simulink model "comparing_controllers"  (R2020a)
settings: Solver=VariableStepAuto  StartTime=0.0  StopTime=50  RelTol=1e-3
libraries: aerolibutil x20, sharedutil x10, slctrlblks x6
(part 2 of 3)

== system comparing_controllers/PD Gravity Compensated Controller/6 DOF PD Gravity Comp Controller/Subsystem3/Subsystem1 ==
  NED : Inport
  Demux : Demux  Outputs=2
  Demux1 : Demux  Outputs=3
  Derivative : Derivative  Commented=on
  Invert 3x3 Matrix : aerolibutil/Invert  3x3 Matrix
  Invert 3x3 Matrix1 : aerolibutil/Invert  3x3 Matrix  Commented=on
  MatrixMultiply : Product  Commented=on  Multiplication=Matrix(*)
  MatrixMultiply1 : Product  Multiplication=Matrix(*)
  Mux1 : Mux  Inputs=3
  Rzxy : Subsystem
  T : Subsystem  Commented=on
  Terminator : Terminator  Commented=on
  pos_body : Outport
  wires:
  Demux1/2 -> Mux1/2, T/2(In2)  "theta"
  Demux1/1 -> Mux1/1, T/1(In1)  "phi"
  Rzxy/1(J) -> Invert 3x3 Matrix/1
  Mux1/1 -> Derivative/1, Rzxy/1(angles)
  Derivative/1 -> MatrixMultiply/2  "euler_dot"
  Invert 3x3 Matrix1/1 -> MatrixMultiply/1  "T'"
  Demux1/3 -> Mux1/3  "psi"
  MatrixMultiply/1 -> Terminator/1  "ang_vel_body"
  T/1(T) -> Invert 3x3 Matrix1/1
  Invert 3x3 Matrix/1 -> MatrixMultiply1/1  "R'"
  MatrixMultiply1/1 -> pos_body/1
  NED/1 -> Demux/1
  Demux/2 -> Demux1/1
  Demux/1 -> MatrixMultiply1/2

== system comparing_controllers/PD Gravity Compensated Controller/6 DOF PD Gravity Comp Controller/Subsystem3/Subsystem2 ==
  NED : Inport
  Demux : Demux  Outputs=2
  Demux1 : Demux  Outputs=3
  Derivative : Derivative  Commented=on
  Invert 3x3 Matrix : aerolibutil/Invert  3x3 Matrix
  Invert 3x3 Matrix1 : aerolibutil/Invert  3x3 Matrix  Commented=on
  MatrixMultiply : Product  Commented=on  Multiplication=Matrix(*)
  MatrixMultiply1 : Product  Multiplication=Matrix(*)
  Mux1 : Mux  Inputs=3
  Rzxy : Subsystem
  T : Subsystem  Commented=on
  Terminator : Terminator  Commented=on
  pos_body : Outport
  wires:
  Demux1/2 -> Mux1/2, T/2(In2)  "theta"
  Demux1/1 -> Mux1/1, T/1(In1)  "phi"
  Rzxy/1(J) -> Invert 3x3 Matrix/1
  Mux1/1 -> Derivative/1, Rzxy/1(angles)
  Derivative/1 -> MatrixMultiply/2  "euler_dot"
  Invert 3x3 Matrix1/1 -> MatrixMultiply/1  "T'"
  Demux1/3 -> Mux1/3  "psi"
  MatrixMultiply/1 -> Terminator/1  "ang_vel_body"
  T/1(T) -> Invert 3x3 Matrix1/1
  Invert 3x3 Matrix/1 -> MatrixMultiply1/1  "R'"
  MatrixMultiply1/1 -> pos_body/1
  NED/1 -> Demux/1
  Demux/2 -> Demux1/1
  Demux/1 -> MatrixMultiply1/2

== system comparing_controllers/PD Gravity Compensated Controller/6 DOF PD Gravity Comp Controller/Transform/Subsystem1 ==
  NED : Inport
  Demux : Demux  Outputs=2
  Demux1 : Demux  Outputs=3
  Derivative : Derivative  Commented=on
  Invert 3x3 Matrix : aerolibutil/Invert  3x3 Matrix
  Invert 3x3 Matrix1 : aerolibutil/Invert  3x3 Matrix  Commented=on
  MatrixMultiply : Product  Commented=on  Multiplication=Matrix(*)
  MatrixMultiply1 : Product  Multiplication=Matrix(*)
  Mux1 : Mux  Inputs=3
  Rzxy : Subsystem
  T : Subsystem  Commented=on
  Terminator : Terminator  Commented=on
  pos_body : Outport
  wires:
  Demux1/2 -> Mux1/2, T/2(In2)  "theta"
  Demux1/1 -> Mux1/1, T/1(In1)  "phi"
  Rzxy/1(J) -> Invert 3x3 Matrix/1
  Mux1/1 -> Derivative/1, Rzxy/1(angles)
  Derivative/1 -> MatrixMultiply/2  "euler_dot"
  Invert 3x3 Matrix1/1 -> MatrixMultiply/1  "T'"
  Demux1/3 -> Mux1/3  "psi"
  MatrixMultiply/1 -> Terminator/1  "ang_vel_body"
  T/1(T) -> Invert 3x3 Matrix1/1
  Invert 3x3 Matrix/1 -> MatrixMultiply1/1  "R'"
  MatrixMultiply1/1 -> pos_body/1
  NED/1 -> Demux/1
  Demux/2 -> Demux1/1
  Demux/1 -> MatrixMultiply1/2

== system comparing_controllers/PD Gravity Compensated Controller/6 DOF PD Gravity Comp Controller/Transform/Subsystem2 ==
  NED : Inport
  Demux : Demux  Outputs=2
  Demux1 : Demux  Outputs=3
  Derivative : Derivative  Commented=on
  Invert 3x3 Matrix : aerolibutil/Invert  3x3 Matrix
  Invert 3x3 Matrix1 : aerolibutil/Invert  3x3 Matrix  Commented=on
  MatrixMultiply : Product  Commented=on  Multiplication=Matrix(*)
  MatrixMultiply1 : Product  Multiplication=Matrix(*)
  Mux1 : Mux  Inputs=3
  Rzxy : Subsystem
  T : Subsystem  Commented=on
  Terminator : Terminator  Commented=on
  pos_body : Outport
  wires:
  Demux1/2 -> Mux1/2, T/2(In2)  "theta"
  Demux1/1 -> Mux1/1, T/1(In1)  "phi"
  Rzxy/1(J) -> Invert 3x3 Matrix/1
  Mux1/1 -> Derivative/1, Rzxy/1(angles)
  Derivative/1 -> MatrixMultiply/2  "euler_dot"
  Invert 3x3 Matrix1/1 -> MatrixMultiply/1  "T'"
  Demux1/3 -> Mux1/3  "psi"
  MatrixMultiply/1 -> Terminator/1  "ang_vel_body"
  T/1(T) -> Invert 3x3 Matrix1/1
  Invert 3x3 Matrix/1 -> MatrixMultiply1/1  "R'"
  MatrixMultiply1/1 -> pos_body/1
  NED/1 -> Demux/1
  Demux/2 -> Demux1/1
  Demux/1 -> MatrixMultiply1/2

== system comparing_controllers/PID Controller/6 DOF PID Controller/Transform/Subsystem1 ==
  NED : Inport
  Demux : Demux  Outputs=2
  Demux1 : Demux  Outputs=3
  Derivative : Derivative  Commented=on
  Invert 3x3 Matrix : aerolibutil/Invert  3x3 Matrix
  Invert 3x3 Matrix1 : aerolibutil/Invert  3x3 Matrix  Commented=on
  MatrixMultiply : Product  Commented=on  Multiplication=Matrix(*)
  MatrixMultiply1 : Product  Multiplication=Matrix(*)
  Mux1 : Mux  Inputs=3
  Rzxy : Subsystem
  T : Subsystem  Commented=on
  Terminator : Terminator  Commented=on
  pos_body : Outport
  wires:
  Demux1/2 -> Mux1/2, T/2(In2)  "theta"
  Demux1/1 -> Mux1/1, T/1(In1)  "phi"
  Rzxy/1(J) -> Invert 3x3 Matrix/1
  Mux1/1 -> Derivative/1, Rzxy/1(angles)
  Derivative/1 -> MatrixMultiply/2  "euler_dot"
  Invert 3x3 Matrix1/1 -> MatrixMultiply/1  "T'"
  Demux1/3 -> Mux1/3  "psi"
  MatrixMultiply/1 -> Terminator/1  "ang_vel_body"
  T/1(T) -> Invert 3x3 Matrix1/1
  Invert 3x3 Matrix/1 -> MatrixMultiply1/1  "R'"
  MatrixMultiply1/1 -> pos_body/1
  NED/1 -> Demux/1
  Demux/2 -> Demux1/1
  Demux/1 -> MatrixMultiply1/2

== system comparing_controllers/PID Controller/6 DOF PID Controller/Transform/Subsystem2 ==
  NED : Inport
  Demux : Demux  Outputs=2
  Demux1 : Demux  Outputs=3
  Derivative : Derivative  Commented=on
  Invert 3x3 Matrix : aerolibutil/Invert  3x3 Matrix
  Invert 3x3 Matrix1 : aerolibutil/Invert  3x3 Matrix  Commented=on
  MatrixMultiply : Product  Commented=on  Multiplication=Matrix(*)
  MatrixMultiply1 : Product  Multiplication=Matrix(*)
  Mux1 : Mux  Inputs=3
  Rzxy : Subsystem
  T : Subsystem  Commented=on
  Terminator : Terminator  Commented=on
  pos_body : Outport
  wires:
  Demux1/2 -> Mux1/2, T/2(In2)  "theta"
  Demux1/1 -> Mux1/1, T/1(In1)  "phi"
  Rzxy/1(J) -> Invert 3x3 Matrix/1
  Mux1/1 -> Derivative/1, Rzxy/1(angles)
  Derivative/1 -> MatrixMultiply/2  "euler_dot"
  Invert 3x3 Matrix1/1 -> MatrixMultiply/1  "T'"
  Demux1/3 -> Mux1/3  "psi"
  MatrixMultiply/1 -> Terminator/1  "ang_vel_body"
  T/1(T) -> Invert 3x3 Matrix1/1
  Invert 3x3 Matrix/1 -> MatrixMultiply1/1  "R'"
  MatrixMultiply1/1 -> pos_body/1
  NED/1 -> Demux/1
  Demux/2 -> Demux1/1
  Demux/1 -> MatrixMultiply1/2

== system comparing_controllers/Computed Torque/Computed Torque Controller/Transform/Subsystem1/Rzxy ==
  angles : Inport
  3-2-1 convention : Product  Inputs=3  Multiplication=Matrix(*)
  Demux : Demux  Outputs=3
  MATLAB Function1 : MATLAB Function  TreatAsAtomicUnit=on
  MATLAB Function2 : MATLAB Function  TreatAsAtomicUnit=on
  MATLAB Function3 : MATLAB Function  TreatAsAtomicUnit=on
  J : Outport
  wires:
  Demux/1 -> MATLAB Function1/1(phi)
  MATLAB Function3/1(Rz) -> 3-2-1 convention/1
  MATLAB Function2/1(Ry) -> 3-2-1 convention/2
  Demux/3 -> MATLAB Function3/1(psi)
  MATLAB Function1/1(Rx) -> 3-2-1 convention/3
  3-2-1 convention/1 -> J/1
  angles/1 -> Demux/1
  Demux/2 -> MATLAB Function2/1(theta)

== system comparing_controllers/Computed Torque/Computed Torque Controller/Transform/Subsystem1/T ==
  In1 : Inport
  In2 : Inport  Port=2
  Constant1 : Constant
  Constant2 : Constant  Value=0
  Create 3x3 Matrix : sharedutil/Create 3x3 Matrix  aMode=aMode
      settings: SourceProductBaseCode=AE,PW,MT,VE,VP
  Divide : Product  Inputs=*/
  Divide1 : Product  Inputs=*/
  Gain : Gain  Gain=-1
  Product : Product
  Product1 : Product
  Sin : Trigonometry
  Sin1 : Trigonometry  Operator=cos
  Sin2 : Trigonometry  Operator=tan
  Sin3 : Trigonometry  Operator=cos
  T : Outport
  wires:
  Constant2/1 -> Create 3x3 Matrix/7, Create 3x3 Matrix/4
  Create 3x3 Matrix/1 -> T/1
  Gain/1 -> Create 3x3 Matrix/6
  Divide1/1 -> Create 3x3 Matrix/9
  Product/1 -> Create 3x3 Matrix/2
  Sin1/1 -> Divide1/1, Create 3x3 Matrix/5, Product1/1
  In1/1 -> Sin1/1, Sin/1  "phi"
  Sin2/1 -> Product/2, Product1/2
  Divide/1 -> Create 3x3 Matrix/8
  Product1/1 -> Create 3x3 Matrix/3
  Sin3/1 -> Divide1/2, Divide/2
  In2/1 -> Sin2/1, Sin3/1  "theta"
  Sin/1 -> Gain/1, Divide/1, Product/1
  Constant1/1 -> Create 3x3 Matrix/1

== system comparing_controllers/Computed Torque/Computed Torque Controller/Transform/Subsystem2/Rzxy ==
  angles : Inport
  3-2-1 convention : Product  Inputs=3  Multiplication=Matrix(*)
  Demux : Demux  Outputs=3
  MATLAB Function1 : MATLAB Function  TreatAsAtomicUnit=on
  MATLAB Function2 : MATLAB Function  TreatAsAtomicUnit=on
  MATLAB Function3 : MATLAB Function  TreatAsAtomicUnit=on
  J : Outport
  wires:
  Demux/1 -> MATLAB Function1/1(phi)
  MATLAB Function3/1(Rz) -> 3-2-1 convention/1
  MATLAB Function2/1(Ry) -> 3-2-1 convention/2
  Demux/3 -> MATLAB Function3/1(psi)
  MATLAB Function1/1(Rx) -> 3-2-1 convention/3
  3-2-1 convention/1 -> J/1
  angles/1 -> Demux/1
  Demux/2 -> MATLAB Function2/1(theta)

== system comparing_controllers/Computed Torque/Computed Torque Controller/Transform/Subsystem2/T ==
  In1 : Inport
  In2 : Inport  Port=2
  Constant1 : Constant
  Constant2 : Constant  Value=0
  Create 3x3 Matrix : sharedutil/Create 3x3 Matrix  aMode=aMode
      settings: SourceProductBaseCode=AE,PW,MT,VE,VP
  Divide : Product  Inputs=*/
  Divide1 : Product  Inputs=*/
  Gain : Gain  Gain=-1
  Product : Product
  Product1 : Product
  Sin : Trigonometry
  Sin1 : Trigonometry  Operator=cos
  Sin2 : Trigonometry  Operator=tan
  Sin3 : Trigonometry  Operator=cos
  T : Outport
  wires:
  Constant2/1 -> Create 3x3 Matrix/7, Create 3x3 Matrix/4
  Create 3x3 Matrix/1 -> T/1
  Gain/1 -> Create 3x3 Matrix/6
  Divide1/1 -> Create 3x3 Matrix/9
  Product/1 -> Create 3x3 Matrix/2
  Sin1/1 -> Divide1/1, Create 3x3 Matrix/5, Product1/1
  In1/1 -> Sin1/1, Sin/1  "phi"
  Sin2/1 -> Product/2, Product1/2
  Divide/1 -> Create 3x3 Matrix/8
  Product1/1 -> Create 3x3 Matrix/3
  Sin3/1 -> Divide1/2, Divide/2
  In2/1 -> Sin2/1, Sin3/1  "theta"
  Sin/1 -> Gain/1, Divide/1, Product/1
  Constant1/1 -> Create 3x3 Matrix/1

== system comparing_controllers/PD Controller/6 DOF PD Controller/Transform/Subsystem1/Rzxy ==
  angles : Inport
  3-2-1 convention : Product  Inputs=3  Multiplication=Matrix(*)
  Demux : Demux  Outputs=3
  MATLAB Function1 : MATLAB Function  TreatAsAtomicUnit=on
  MATLAB Function2 : MATLAB Function  TreatAsAtomicUnit=on
  MATLAB Function3 : MATLAB Function  TreatAsAtomicUnit=on
  J : Outport
  wires:
  Demux/1 -> MATLAB Function1/1(phi)
  MATLAB Function3/1(Rz) -> 3-2-1 convention/1
  MATLAB Function2/1(Ry) -> 3-2-1 convention/2
  Demux/3 -> MATLAB Function3/1(psi)
  MATLAB Function1/1(Rx) -> 3-2-1 convention/3
  3-2-1 convention/1 -> J/1
  angles/1 -> Demux/1
  Demux/2 -> MATLAB Function2/1(theta)

== system comparing_controllers/PD Controller/6 DOF PD Controller/Transform/Subsystem1/T ==
  In1 : Inport
  In2 : Inport  Port=2
  Constant1 : Constant
  Constant2 : Constant  Value=0
  Create 3x3 Matrix : sharedutil/Create 3x3 Matrix  aMode=aMode
      settings: SourceProductBaseCode=AE,PW,MT,VE,VP
  Divide : Product  Inputs=*/
  Divide1 : Product  Inputs=*/
  Gain : Gain  Gain=-1
  Product : Product
  Product1 : Product
  Sin : Trigonometry
  Sin1 : Trigonometry  Operator=cos
  Sin2 : Trigonometry  Operator=tan
  Sin3 : Trigonometry  Operator=cos
  T : Outport
  wires:
  Constant2/1 -> Create 3x3 Matrix/7, Create 3x3 Matrix/4
  Create 3x3 Matrix/1 -> T/1
  Gain/1 -> Create 3x3 Matrix/6
  Divide1/1 -> Create 3x3 Matrix/9
  Product/1 -> Create 3x3 Matrix/2
  Sin1/1 -> Divide1/1, Create 3x3 Matrix/5, Product1/1
  In1/1 -> Sin1/1, Sin/1  "phi"
  Sin2/1 -> Product/2, Product1/2
  Divide/1 -> Create 3x3 Matrix/8
  Product1/1 -> Create 3x3 Matrix/3
  Sin3/1 -> Divide1/2, Divide/2
  In2/1 -> Sin2/1, Sin3/1  "theta"
  Sin/1 -> Gain/1, Divide/1, Product/1
  Constant1/1 -> Create 3x3 Matrix/1

== system comparing_controllers/PD Controller/6 DOF PD Controller/Transform/Subsystem2/Rzxy ==
  angles : Inport
  3-2-1 convention : Product  Inputs=3  Multiplication=Matrix(*)
  Demux : Demux  Outputs=3
  MATLAB Function1 : MATLAB Function  TreatAsAtomicUnit=on
  MATLAB Function2 : MATLAB Function  TreatAsAtomicUnit=on
  MATLAB Function3 : MATLAB Function  TreatAsAtomicUnit=on
  J : Outport
  wires:
  Demux/1 -> MATLAB Function1/1(phi)
  MATLAB Function3/1(Rz) -> 3-2-1 convention/1
  MATLAB Function2/1(Ry) -> 3-2-1 convention/2
  Demux/3 -> MATLAB Function3/1(psi)
  MATLAB Function1/1(Rx) -> 3-2-1 convention/3
  3-2-1 convention/1 -> J/1
  angles/1 -> Demux/1
  Demux/2 -> MATLAB Function2/1(theta)

== system comparing_controllers/PD Controller/6 DOF PD Controller/Transform/Subsystem2/T ==
  In1 : Inport
  In2 : Inport  Port=2
  Constant1 : Constant
  Constant2 : Constant  Value=0
  Create 3x3 Matrix : sharedutil/Create 3x3 Matrix  aMode=aMode
      settings: SourceProductBaseCode=AE,PW,MT,VE,VP
  Divide : Product  Inputs=*/
  Divide1 : Product  Inputs=*/
  Gain : Gain  Gain=-1
  Product : Product
  Product1 : Product
  Sin : Trigonometry
  Sin1 : Trigonometry  Operator=cos
  Sin2 : Trigonometry  Operator=tan
  Sin3 : Trigonometry  Operator=cos
  T : Outport
  wires:
  Constant2/1 -> Create 3x3 Matrix/7, Create 3x3 Matrix/4
  Create 3x3 Matrix/1 -> T/1
  Gain/1 -> Create 3x3 Matrix/6
  Divide1/1 -> Create 3x3 Matrix/9
  Product/1 -> Create 3x3 Matrix/2
  Sin1/1 -> Divide1/1, Create 3x3 Matrix/5, Product1/1
  In1/1 -> Sin1/1, Sin/1  "phi"
  Sin2/1 -> Product/2, Product1/2
  Divide/1 -> Create 3x3 Matrix/8
  Product1/1 -> Create 3x3 Matrix/3
  Sin3/1 -> Divide1/2, Divide/2
  In2/1 -> Sin2/1, Sin3/1  "theta"
  Sin/1 -> Gain/1, Divide/1, Product/1
  Constant1/1 -> Create 3x3 Matrix/1

== system comparing_controllers/PD Gravity Compensated Controller/6 DOF PD Gravity Comp Controller/Subsystem3/Subsystem1/Rzxy ==
  angles : Inport
  3-2-1 convention : Product  Inputs=3  Multiplication=Matrix(*)
  Demux : Demux  Outputs=3
  MATLAB Function1 : MATLAB Function  TreatAsAtomicUnit=on
  MATLAB Function2 : MATLAB Function  TreatAsAtomicUnit=on
  MATLAB Function3 : MATLAB Function  TreatAsAtomicUnit=on
  J : Outport
  wires:
  Demux/1 -> MATLAB Function1/1(phi)
  MATLAB Function3/1(Rz) -> 3-2-1 convention/1
  MATLAB Function2/1(Ry) -> 3-2-1 convention/2
  Demux/3 -> MATLAB Function3/1(psi)
  MATLAB Function1/1(Rx) -> 3-2-1 convention/3
  3-2-1 convention/1 -> J/1
  angles/1 -> Demux/1
  Demux/2 -> MATLAB Function2/1(theta)

== system comparing_controllers/PD Gravity Compensated Controller/6 DOF PD Gravity Comp Controller/Subsystem3/Subsystem1/T ==
  In1 : Inport
  In2 : Inport  Port=2
  Constant1 : Constant
  Constant2 : Constant  Value=0
  Create 3x3 Matrix : sharedutil/Create 3x3 Matrix  aMode=aMode
      settings: SourceProductBaseCode=AE,PW,MT,VE,VP
  Divide : Product  Inputs=*/
  Divide1 : Product  Inputs=*/
  Gain : Gain  Gain=-1
  Product : Product
  Product1 : Product
  Sin : Trigonometry
  Sin1 : Trigonometry  Operator=cos
  Sin2 : Trigonometry  Operator=tan
  Sin3 : Trigonometry  Operator=cos
  T : Outport
  wires:
  Constant2/1 -> Create 3x3 Matrix/7, Create 3x3 Matrix/4
  Create 3x3 Matrix/1 -> T/1
  Gain/1 -> Create 3x3 Matrix/6
  Divide1/1 -> Create 3x3 Matrix/9
  Product/1 -> Create 3x3 Matrix/2
  Sin1/1 -> Divide1/1, Create 3x3 Matrix/5, Product1/1
  In1/1 -> Sin1/1, Sin/1  "phi"
  Sin2/1 -> Product/2, Product1/2
  Divide/1 -> Create 3x3 Matrix/8
  Product1/1 -> Create 3x3 Matrix/3
  Sin3/1 -> Divide1/2, Divide/2
  In2/1 -> Sin2/1, Sin3/1  "theta"
  Sin/1 -> Gain/1, Divide/1, Product/1
  Constant1/1 -> Create 3x3 Matrix/1

== system comparing_controllers/PD Gravity Compensated Controller/6 DOF PD Gravity Comp Controller/Subsystem3/Subsystem2/Rzxy ==
  angles : Inport
  3-2-1 convention : Product  Inputs=3  Multiplication=Matrix(*)
  Demux : Demux  Outputs=3
  MATLAB Function1 : MATLAB Function  TreatAsAtomicUnit=on
  MATLAB Function2 : MATLAB Function  TreatAsAtomicUnit=on
  MATLAB Function3 : MATLAB Function  TreatAsAtomicUnit=on
  J : Outport
  wires:
  Demux/1 -> MATLAB Function1/1(phi)
  MATLAB Function3/1(Rz) -> 3-2-1 convention/1
  MATLAB Function2/1(Ry) -> 3-2-1 convention/2
  Demux/3 -> MATLAB Function3/1(psi)
  MATLAB Function1/1(Rx) -> 3-2-1 convention/3
  3-2-1 convention/1 -> J/1
  angles/1 -> Demux/1
  Demux/2 -> MATLAB Function2/1(theta)

== system comparing_controllers/PD Gravity Compensated Controller/6 DOF PD Gravity Comp Controller/Subsystem3/Subsystem2/T ==
  In1 : Inport
  In2 : Inport  Port=2
  Constant1 : Constant
  Constant2 : Constant  Value=0
  Create 3x3 Matrix : sharedutil/Create 3x3 Matrix  aMode=aMode
      settings: SourceProductBaseCode=AE,PW,MT,VE,VP
  Divide : Product  Inputs=*/
  Divide1 : Product  Inputs=*/
  Gain : Gain  Gain=-1
  Product : Product
  Product1 : Product
  Sin : Trigonometry
  Sin1 : Trigonometry  Operator=cos
  Sin2 : Trigonometry  Operator=tan
  Sin3 : Trigonometry  Operator=cos
  T : Outport
  wires:
  Constant2/1 -> Create 3x3 Matrix/7, Create 3x3 Matrix/4
  Create 3x3 Matrix/1 -> T/1
  Gain/1 -> Create 3x3 Matrix/6
  Divide1/1 -> Create 3x3 Matrix/9
  Product/1 -> Create 3x3 Matrix/2
  Sin1/1 -> Divide1/1, Create 3x3 Matrix/5, Product1/1
  In1/1 -> Sin1/1, Sin/1  "phi"
  Sin2/1 -> Product/2, Product1/2
  Divide/1 -> Create 3x3 Matrix/8
  Product1/1 -> Create 3x3 Matrix/3
  Sin3/1 -> Divide1/2, Divide/2
  In2/1 -> Sin2/1, Sin3/1  "theta"
  Sin/1 -> Gain/1, Divide/1, Product/1
  Constant1/1 -> Create 3x3 Matrix/1

== system comparing_controllers/PD Gravity Compensated Controller/6 DOF PD Gravity Comp Controller/Transform/Subsystem1/Rzxy ==
  angles : Inport
  3-2-1 convention : Product  Inputs=3  Multiplication=Matrix(*)
  Demux : Demux  Outputs=3
  MATLAB Function1 : MATLAB Function  TreatAsAtomicUnit=on
  MATLAB Function2 : MATLAB Function  TreatAsAtomicUnit=on
  MATLAB Function3 : MATLAB Function  TreatAsAtomicUnit=on
  J : Outport
  wires:
  Demux/1 -> MATLAB Function1/1(phi)
  MATLAB Function3/1(Rz) -> 3-2-1 convention/1
  MATLAB Function2/1(Ry) -> 3-2-1 convention/2
  Demux/3 -> MATLAB Function3/1(psi)
  MATLAB Function1/1(Rx) -> 3-2-1 convention/3
  3-2-1 convention/1 -> J/1
  angles/1 -> Demux/1
  Demux/2 -> MATLAB Function2/1(theta)

== system comparing_controllers/PD Gravity Compensated Controller/6 DOF PD Gravity Comp Controller/Transform/Subsystem1/T ==
  In1 : Inport
  In2 : Inport  Port=2
  Constant1 : Constant
  Constant2 : Constant  Value=0
  Create 3x3 Matrix : sharedutil/Create 3x3 Matrix  aMode=aMode
      settings: SourceProductBaseCode=AE,PW,MT,VE,VP
  Divide : Product  Inputs=*/
  Divide1 : Product  Inputs=*/
  Gain : Gain  Gain=-1
  Product : Product
  Product1 : Product
  Sin : Trigonometry
  Sin1 : Trigonometry  Operator=cos
  Sin2 : Trigonometry  Operator=tan
  Sin3 : Trigonometry  Operator=cos
  T : Outport
  wires:
  Constant2/1 -> Create 3x3 Matrix/7, Create 3x3 Matrix/4
  Create 3x3 Matrix/1 -> T/1
  Gain/1 -> Create 3x3 Matrix/6
  Divide1/1 -> Create 3x3 Matrix/9
  Product/1 -> Create 3x3 Matrix/2
  Sin1/1 -> Divide1/1, Create 3x3 Matrix/5, Product1/1
  In1/1 -> Sin1/1, Sin/1  "phi"
  Sin2/1 -> Product/2, Product1/2
  Divide/1 -> Create 3x3 Matrix/8
  Product1/1 -> Create 3x3 Matrix/3
  Sin3/1 -> Divide1/2, Divide/2
  In2/1 -> Sin2/1, Sin3/1  "theta"
  Sin/1 -> Gain/1, Divide/1, Product/1
  Constant1/1 -> Create 3x3 Matrix/1

== system comparing_controllers/PD Gravity Compensated Controller/6 DOF PD Gravity Comp Controller/Transform/Subsystem2/Rzxy ==
  angles : Inport
  3-2-1 convention : Product  Inputs=3  Multiplication=Matrix(*)
  Demux : Demux  Outputs=3
  MATLAB Function1 : MATLAB Function  TreatAsAtomicUnit=on
  MATLAB Function2 : MATLAB Function  TreatAsAtomicUnit=on
  MATLAB Function3 : MATLAB Function  TreatAsAtomicUnit=on
  J : Outport
  wires:
  Demux/1 -> MATLAB Function1/1(phi)
  MATLAB Function3/1(Rz) -> 3-2-1 convention/1
  MATLAB Function2/1(Ry) -> 3-2-1 convention/2
  Demux/3 -> MATLAB Function3/1(psi)
  MATLAB Function1/1(Rx) -> 3-2-1 convention/3
  3-2-1 convention/1 -> J/1
  angles/1 -> Demux/1
  Demux/2 -> MATLAB Function2/1(theta)

== system comparing_controllers/PD Gravity Compensated Controller/6 DOF PD Gravity Comp Controller/Transform/Subsystem2/T ==
  In1 : Inport
  In2 : Inport  Port=2
  Constant1 : Constant
  Constant2 : Constant  Value=0
  Create 3x3 Matrix : sharedutil/Create 3x3 Matrix  aMode=aMode
      settings: SourceProductBaseCode=AE,PW,MT,VE,VP
  Divide : Product  Inputs=*/
  Divide1 : Product  Inputs=*/
  Gain : Gain  Gain=-1
  Product : Product
  Product1 : Product
  Sin : Trigonometry
  Sin1 : Trigonometry  Operator=cos
  Sin2 : Trigonometry  Operator=tan
  Sin3 : Trigonometry  Operator=cos
  T : Outport
  wires:
  Constant2/1 -> Create 3x3 Matrix/7, Create 3x3 Matrix/4
  Create 3x3 Matrix/1 -> T/1
  Gain/1 -> Create 3x3 Matrix/6
  Divide1/1 -> Create 3x3 Matrix/9
  Product/1 -> Create 3x3 Matrix/2
  Sin1/1 -> Divide1/1, Create 3x3 Matrix/5, Product1/1
  In1/1 -> Sin1/1, Sin/1  "phi"
  Sin2/1 -> Product/2, Product1/2
  Divide/1 -> Create 3x3 Matrix/8
  Product1/1 -> Create 3x3 Matrix/3
  Sin3/1 -> Divide1/2, Divide/2
  In2/1 -> Sin2/1, Sin3/1  "theta"
  Sin/1 -> Gain/1, Divide/1, Product/1
  Constant1/1 -> Create 3x3 Matrix/1

== system comparing_controllers/PID Controller/6 DOF PID Controller/Transform/Subsystem1/Rzxy ==
  angles : Inport
  3-2-1 convention : Product  Inputs=3  Multiplication=Matrix(*)
  Demux : Demux  Outputs=3
  MATLAB Function1 : MATLAB Function  TreatAsAtomicUnit=on
  MATLAB Function2 : MATLAB Function  TreatAsAtomicUnit=on
  MATLAB Function3 : MATLAB Function  TreatAsAtomicUnit=on
  J : Outport
  wires:
  Demux/1 -> MATLAB Function1/1(phi)
  MATLAB Function3/1(Rz) -> 3-2-1 convention/1
  MATLAB Function2/1(Ry) -> 3-2-1 convention/2
  Demux/3 -> MATLAB Function3/1(psi)
  MATLAB Function1/1(Rx) -> 3-2-1 convention/3
  3-2-1 convention/1 -> J/1
  angles/1 -> Demux/1
  Demux/2 -> MATLAB Function2/1(theta)

== system comparing_controllers/PID Controller/6 DOF PID Controller/Transform/Subsystem1/T ==
  In1 : Inport
  In2 : Inport  Port=2
  Constant1 : Constant
  Constant2 : Constant  Value=0
  Create 3x3 Matrix : sharedutil/Create 3x3 Matrix  aMode=aMode
      settings: SourceProductBaseCode=AE,PW,MT,VE,VP
  Divide : Product  Inputs=*/
  Divide1 : Product  Inputs=*/
  Gain : Gain  Gain=-1
  Product : Product
  Product1 : Product
  Sin : Trigonometry
  Sin1 : Trigonometry  Operator=cos
  Sin2 : Trigonometry  Operator=tan
  Sin3 : Trigonometry  Operator=cos
  T : Outport
  wires:
  Constant2/1 -> Create 3x3 Matrix/7, Create 3x3 Matrix/4
  Create 3x3 Matrix/1 -> T/1
  Gain/1 -> Create 3x3 Matrix/6
  Divide1/1 -> Create 3x3 Matrix/9
  Product/1 -> Create 3x3 Matrix/2
  Sin1/1 -> Divide1/1, Create 3x3 Matrix/5, Product1/1
  In1/1 -> Sin1/1, Sin/1  "phi"
  Sin2/1 -> Product/2, Product1/2
  Divide/1 -> Create 3x3 Matrix/8
  Product1/1 -> Create 3x3 Matrix/3
  Sin3/1 -> Divide1/2, Divide/2
  In2/1 -> Sin2/1, Sin3/1  "theta"
  Sin/1 -> Gain/1, Divide/1, Product/1
  Constant1/1 -> Create 3x3 Matrix/1

== system comparing_controllers/PID Controller/6 DOF PID Controller/Transform/Subsystem2/Rzxy ==
  angles : Inport
  3-2-1 convention : Product  Inputs=3  Multiplication=Matrix(*)
  Demux : Demux  Outputs=3
  MATLAB Function1 : MATLAB Function  TreatAsAtomicUnit=on
  MATLAB Function2 : MATLAB Function  TreatAsAtomicUnit=on
  MATLAB Function3 : MATLAB Function  TreatAsAtomicUnit=on
  J : Outport
  wires:
  Demux/1 -> MATLAB Function1/1(phi)
  MATLAB Function3/1(Rz) -> 3-2-1 convention/1
  MATLAB Function2/1(Ry) -> 3-2-1 convention/2
  Demux/3 -> MATLAB Function3/1(psi)
  MATLAB Function1/1(Rx) -> 3-2-1 convention/3
  3-2-1 convention/1 -> J/1
  angles/1 -> Demux/1
  Demux/2 -> MATLAB Function2/1(theta)

== system comparing_controllers/PID Controller/6 DOF PID Controller/Transform/Subsystem2/T ==
  In1 : Inport
  In2 : Inport  Port=2
  Constant1 : Constant
  Constant2 : Constant  Value=0
  Create 3x3 Matrix : sharedutil/Create 3x3 Matrix  aMode=aMode
      settings: SourceProductBaseCode=AE,PW,MT,VE,VP
  Divide : Product  Inputs=*/
  Divide1 : Product  Inputs=*/
  Gain : Gain  Gain=-1
  Product : Product
  Product1 : Product
  Sin : Trigonometry
  Sin1 : Trigonometry  Operator=cos
  Sin2 : Trigonometry  Operator=tan
  Sin3 : Trigonometry  Operator=cos
  T : Outport
  wires:
  Constant2/1 -> Create 3x3 Matrix/7, Create 3x3 Matrix/4
  Create 3x3 Matrix/1 -> T/1
  Gain/1 -> Create 3x3 Matrix/6
  Divide1/1 -> Create 3x3 Matrix/9
  Product/1 -> Create 3x3 Matrix/2
  Sin1/1 -> Divide1/1, Create 3x3 Matrix/5, Product1/1
  In1/1 -> Sin1/1, Sin/1  "phi"
  Sin2/1 -> Product/2, Product1/2
  Divide/1 -> Create 3x3 Matrix/8
  Product1/1 -> Create 3x3 Matrix/3
  Sin3/1 -> Divide1/2, Divide/2
  In2/1 -> Sin2/1, Sin3/1  "theta"
  Sin/1 -> Gain/1, Divide/1, Product/1
  Constant1/1 -> Create 3x3 Matrix/1

== matlab function comparing_controllers/PD Controller/6 DOF PD Controller/Transform/Subsystem1/Rzxy/MATLAB Function2 ==
  data: theta input; Ry output
function Ry = Ry(theta)
Ry = [ cos(theta) 0 sin(theta);
       0          1     0 ;
       -sin(theta) 0 cos(theta); ];

== matlab function comparing_controllers/PD Controller/6 DOF PD Controller/Transform/Subsystem1/Rzxy/MATLAB Function3 ==
  data: psi input; Rz output
function Rz = Rz(psi)
Rz = [ cos(psi) -sin(psi) 0;
       sin(psi) cos(psi)  0;
       0        0         1];

== matlab function comparing_controllers/PD Controller/6 DOF PD Controller/Thrust allocation/MATLAB Function1 ==
  data: tau input; thrust output; alpha input; rx_v input; ry_v input; unused input; rx_h input; ry_h input; rz_h input
function thrust = thrust_allocation(tau, alpha, rx_v, ry_v, ~, rx_h, ry_h, rz_h)
% Mapping matrix
T = [cos(alpha) cos(alpha) -cos(alpha) -cos(alpha) 0 0;
     -sin(alpha) sin(alpha) -sin(alpha) sin(alpha) 0 0;
     0 0 0 0 -1 -1;
     -sin(alpha)*rz_h sin(alpha)*rz_h -sin(alpha)*rz_h sin(alpha)*rz_h -ry_v ry_v;
     -cos(alpha)*rz_h -cos(alpha)*rz_h cos(alpha)*rz_h cos(alpha)*rz_h -rx_v rx_v;
     -(rx_h*sin(alpha)+ry_h*cos(alpha)) (rx_h*sin(alpha)+ry_h*cos(alpha)) (rx_h*sin(alpha)+ry_h*cos(alpha)) -(rx_h*sin(alpha)+ry_h*cos(alpha)) 0 0
    ];
% Control input with Moore–Penrose pseudo-inverse
thrust = pinv(T)*tau;

== matlab function comparing_controllers/PD Gravity Compensated Controller/6 DOF PD Gravity Comp Controller/6 PD Gravity Comp Controllers/MATLAB Function1 ==
  data: phi input; theta input; g_eta output; unused input
function g_eta = g_eta(phi, theta, ~)
%Fossen (2011): According to (2.2), the sign of the restoring forces and moments fbi 
%and mbi = rbi × fbi , i ∈ {g, b}, must be changed when moving these terms to the 
%left-hand side of (2.2) that is the vector g(η). Pag 60 Handbook of ...

r_g = [0 0 0].';    % Distance from origin to center of mass
r_b = [0 0 -0.10726].';    % Distance from origin to center of buoyancy
m = 24;
W = m*9.81;
B = W*1.005; 
% Restoring forces
g_eta = [ (W-B)*sin(theta);
          -(W-B)*cos(theta)*sin(phi);
          -(W-B)*cos(theta)*cos(phi);
          -(r_g(2)*W-r_b(2)*B)*cos(theta)*cos(phi) + (r_g(3)*W-r_b(3)*B)*cos(theta)*sin(phi);
           (r_g(3)*W-r_b(3)*B)*sin(theta)             + (r_g(1)*W-r_b(1)*B)*cos(theta)*cos(phi)
          -(r_g(1)*W-r_b(1)*B)*cos(theta)*sin(phi) - (r_g(2)*W-r_b(2)*B)*sin(theta)          ];

== matlab function comparing_controllers/PD Gravity Compensated Controller/6 DOF PD Gravity Comp Controller/Subsystem/MATLAB Function ==
  data: thrust input; tau output; theta input; rx_v input; ry_v input; unused input; rx_h input; ry_h input; rz_h input
function tau = thrust_conversion(thrust, theta, rx_v, ry_v, ~, rx_h, ry_h, rz_h)
% Errores numericos. El input esta saturado a [100,-100], y estas salidas
% dan valores muchisimo mayores a 35 N c/u
tau = [0 0 0 0 0 0].';
% For surge
s_val = thrust(1)/cos(theta)/4;
tau(1) = tau(1)+s_val;
tau(2) = tau(2)+s_val;
tau(3) = tau(3)-s_val;
tau(4) = tau(4)-s_val;

% For sway
sw_val = thrust(2)/sin(theta)/4;
tau(1) = tau(1)-sw_val;
tau(2) = tau(2)+sw_val;
tau(3) = tau(3)-sw_val;
tau(4) = tau(4)+sw_val;

% For heave
tau(5) = tau(5)+(-thrust(3)/2);
tau(6) = tau(6)+(-thrust(3)/2);

% For yaw
y_val = thrust(6)/(rx_h*sin(theta)+ry_h*cos(theta))/4;
tau(1) = tau(1)-y_val;
tau(2) = tau(2)+y_val;
tau(3) = tau(3)+y_val;
tau(4) = tau(4)-y_val;

% K and M come as zero
% For K
if  thrust(4)~= 0
    %disp("K")
    k_val = (thrust(4)-(-tau(1)+tau(2)-tau(3)+tau(4))*sin(theta)*rz_h)/(2*ry_v);
    tau(5) = tau(5)-k_val;
    tau(6) = tau(6)+k_val;
end

% For M
if thrust(5) ~= 0
    %disp("M")
    M_val = (thrust(5)-(-tau(1)-tau(2)+tau(3)+tau(4))*cos(theta)*rz_h)/(2*rx_v);
    tau(5) = tau(5)-M_val;
    tau(6) = tau(6)+M_val;
end
disp(tau)

== matlab function comparing_controllers/PD Gravity Compensated Controller/6 DOF PD Gravity Comp Controller/Subsystem3/Subsystem1/Rzxy/MATLAB Function1 ==
  data: phi input; Rx output
function Rx = Rx(phi)
Rx = [ 1 0 0;
       0 cos(phi) -sin(phi);
       0 sin(phi) cos(phi); ];

== matlab function comparing_controllers/PD Gravity Compensated Controller/6 DOF PD Gravity Comp Controller/Subsystem3/Subsystem1/Rzxy/MATLAB Function2 ==
  data: theta input; Ry output
function Ry = Ry(theta)
Ry = [ cos(theta) 0 sin(theta);
       0          1     0 ;
       -sin(theta) 0 cos(theta); ];

== matlab function comparing_controllers/PD Gravity Compensated Controller/6 DOF PD Gravity Comp Controller/Subsystem3/Subsystem1/Rzxy/MATLAB Function3 ==
  data: psi input; Rz output
function Rz = Rz(psi)
Rz = [ cos(psi) -sin(psi) 0;
       sin(psi) cos(psi)  0;
       0        0         1];

== matlab function comparing_controllers/PD Gravity Compensated Controller/6 DOF PD Gravity Comp Controller/Subsystem3/Subsystem2/Rzxy/MATLAB Function1 ==
  data: phi input; Rx output
function Rx = Rx(phi)
Rx = [ 1 0 0;
       0 cos(phi) -sin(phi);
       0 sin(phi) cos(phi); ];

== matlab function comparing_controllers/PD Gravity Compensated Controller/6 DOF PD Gravity Comp Controller/Subsystem3/Subsystem2/Rzxy/MATLAB Function2 ==
  data: theta input; Ry output
function Ry = Ry(theta)
Ry = [ cos(theta) 0 sin(theta);
       0          1     0 ;
       -sin(theta) 0 cos(theta); ];

== matlab function comparing_controllers/PD Gravity Compensated Controller/6 DOF PD Gravity Comp Controller/Subsystem3/Subsystem2/Rzxy/MATLAB Function3 ==
  data: psi input; Rz output
function Rz = Rz(psi)
Rz = [ cos(psi) -sin(psi) 0;
       sin(psi) cos(psi)  0;
       0        0         1];

== matlab function comparing_controllers/PD Gravity Compensated Controller/6 DOF PD Gravity Comp Controller/Thrust allocation/MATLAB Function ==
  data: thrust input; tau output; theta input; rx_v input; ry_v input; unused input; rx_h input; ry_h input; rz_h input
function tau = thrust_conversion(thrust, theta, rx_v, ry_v, ~, rx_h, ry_h, rz_h)
% Errores numericos. El input esta saturado a [100,-100], y estas salidas
% dan valores muchisimo mayores a 35 N c/u
tau = [0 0 0 0 0 0].';
% For surge
s_val = thrust(1)/cos(theta)/4;
tau(1) = tau(1)+s_val;
tau(2) = tau(2)+s_val;
tau(3) = tau(3)-s_val;
tau(4) = tau(4)-s_val;

% For sway
sw_val = thrust(2)/sin(theta)/4;
tau(1) = tau(1)-sw_val;
tau(2) = tau(2)+sw_val;
tau(3) = tau(3)-sw_val;
tau(4) = tau(4)+sw_val;

% For heave
tau(5) = tau(5)+(-thrust(3)/2);
tau(6) = tau(6)+(-thrust(3)/2);

% For yaw
y_val = thrust(6)/(rx_h*sin(theta)+ry_h*cos(theta))/4;
tau(1) = tau(1)-y_val;
tau(2) = tau(2)+y_val;
tau(3) = tau(3)+y_val;
tau(4) = tau(4)-y_val;

% K and M come as zero
% For K
if  thrust(4)~= 0
    %disp("K")
    k_val = (thrust(4)-(-tau(1)+tau(2)-tau(3)+tau(4))*sin(theta)*rz_h)/(2*ry_v);
    tau(5) = tau(5)-k_val;
    tau(6) = tau(6)+k_val;
end

% For M
if thrust(5) ~= 0
    %disp("M")
    M_val = (thrust(5)-(-tau(1)-tau(2)+tau(3)+tau(4))*cos(theta)*rz_h)/(2*rx_v);
    tau(5) = tau(5)-M_val;
    tau(6) = tau(6)+M_val;
end
disp(tau)

== matlab function comparing_controllers/PD Gravity Compensated Controller/6 DOF PD Gravity Comp Controller/Thrust allocation/MATLAB Function1 ==
  data: tau input; thrust output; alpha input; rx_v input; ry_v input; unused input; rx_h input; ry_h input; rz_h input
function thrust = thrust_allocation(tau, alpha, rx_v, ry_v, ~, rx_h, ry_h, rz_h)
% Mapping matrix
T = [cos(alpha) cos(alpha) -cos(alpha) -cos(alpha) 0 0;
     -sin(alpha) sin(alpha) -sin(alpha) sin(alpha) 0 0;
     0 0 0 0 -1 -1;
     -sin(alpha)*rz_h sin(alpha)*rz_h -sin(alpha)*rz_h sin(alpha)*rz_h -ry_v ry_v;
     -cos(alpha)*rz_h -cos(alpha)*rz_h cos(alpha)*rz_h cos(alpha)*rz_h -rx_v rx_v;
     -(rx_h*sin(alpha)+ry_h*cos(alpha)) (rx_h*sin(alpha)+ry_h*cos(alpha)) (rx_h*sin(alpha)+ry_h*cos(alpha)) -(rx_h*sin(alpha)+ry_h*cos(alpha)) 0 0
    ];
% Control input with Moore–Penrose pseudo-inverse
thrust = pinv(T)*tau;

== matlab function comparing_controllers/PD Gravity Compensated Controller/6 DOF PD Gravity Comp Controller/Transform/Subsystem1/Rzxy/MATLAB Function1 ==
  data: phi input; Rx output
function Rx = Rx(phi)
Rx = [ 1 0 0;
       0 cos(phi) -sin(phi);
       0 sin(phi) cos(phi); ];

== matlab function comparing_controllers/PD Gravity Compensated Controller/6 DOF PD Gravity Comp Controller/Transform/Subsystem1/Rzxy/MATLAB Function2 ==
  data: theta input; Ry output
function Ry = Ry(theta)
Ry = [ cos(theta) 0 sin(theta);
       0          1     0 ;
       -sin(theta) 0 cos(theta); ];

== matlab function comparing_controllers/PD Gravity Compensated Controller/6 DOF PD Gravity Comp Controller/Transform/Subsystem1/Rzxy/MATLAB Function3 ==
  data: psi input; Rz output
function Rz = Rz(psi)
Rz = [ cos(psi) -sin(psi) 0;
       sin(psi) cos(psi)  0;
       0        0         1];

== matlab function comparing_controllers/PD Gravity Compensated Controller/6 DOF PD Gravity Comp Controller/Transform/Subsystem2/Rzxy/MATLAB Function1 ==
  data: phi input; Rx output
function Rx = Rx(phi)
Rx = [ 1 0 0;
       0 cos(phi) -sin(phi);
       0 sin(phi) cos(phi); ];

== matlab function comparing_controllers/PD Gravity Compensated Controller/6 DOF PD Gravity Comp Controller/Transform/Subsystem2/Rzxy/MATLAB Function2 ==
  data: theta input; Ry output
function Ry = Ry(theta)
Ry = [ cos(theta) 0 sin(theta);
       0          1     0 ;
       -sin(theta) 0 cos(theta); ];

== matlab function comparing_controllers/PD Gravity Compensated Controller/6 DOF PD Gravity Comp Controller/Transform/Subsystem2/Rzxy/MATLAB Function3 ==
  data: psi input; Rz output
function Rz = Rz(psi)
Rz = [ cos(psi) -sin(psi) 0;
       sin(psi) cos(psi)  0;
       0        0         1];

== matlab function comparing_controllers/PD Gravity Compensated Controller/UUV 6DOF Model/+-pi ==
  data: NED input; NED output
function NED = check_angles(NED)
% Correct
if abs(NED(4)) > pi 
    NED(4) = (NED(4)/abs(NED(4)))*(abs(NED(4))-2*pi);
end
if abs(NED(5)) > pi 
    NED(5) = (NED(5)/abs(NED(5)))*(abs(NED(5))-2*pi);
end
if abs(NED(6)) > pi
    NED(6) = (NED(6)/abs(NED(6)))*(abs(NED(6))-2*pi);
    disp((NED(6)/abs(NED(6)))*(abs(NED(6))-2*pi))
end

== matlab function comparing_controllers/PD Gravity Compensated Controller/UUV 6DOF Model/MATLAB Function ==
  data: vel_dot output; tau input; vel input; phi input; theta input; NED_dot output; psi input
function [vel_dot,NED_dot]= UUV_forward_dynamics(tau,vel,phi,theta,psi)
% Skew symmetric matrix
S = @(s) [0    -s(3) s(2);
          s(3) 0     -s(1);
          -s(2) s(1)  0    ];  

% Vehicle parameters
m = 24;
vol = 0.02306187;
W = m*9.81;
B = W*1.005; %1000*9.81*vol;

r_g = [0 0 0].';    % Distance from origin to center of mass
r_b = [0 0 -0.10726].';    % Distance from origin to center of buoyancy
I_g = [0.900121387  -0.000186482 0.0072251;
       -0.000186482 1.754494427  0.020319615;
       0.0072251    0.020319615  1.43389     ]; % Rigid-body inertia matrix

% Rigid-Body Inertia Matrix
M_rb = [ m*eye(3)    -m*S(r_g);
         m*S(r_g)         I_g ];

% Added mass matrix
M_a = diag([16.8374 20.2748 35.3180 0.2165 0.6869 0.6157]);

% Mass matrix
M = M_rb + M_a;

% Linear damping coefficients
X_u = -0.3431;
Y_v = 0.0518;
Z_w = -0.5841;
K_p = 0.0064;
M_q = 0.04;
N_r = -0.1063;

D_lin = -diag([X_u Y_v Z_w K_p M_q N_r]);

% Cuadratic damping coefficients
X_uu = -111.7397;
Y_vv = -44.4058;
Z_ww = -157.1951;
K_pp = -0.4634;
M_qq = -0.2902;
N_rr = -2.2897;

%------------ UUV dynamic model parametrization ----------------%
% Rigid-body Coriolis-centripetal Matrix
C_rb = [ zeros(3)             -m*S(vel(1:3))-m*S(vel(4:6))*S(r_g);
        -m*S(vel(1:3))+m*S(r_g)*S(vel(4:6))            -S(I_g*vel(4:6))];

% Coreolis added mass matrix 
C_a = [ 0 0 0   0 -M_a(3,3)*vel(3) M_a(2,2)*vel(2) ;
        0 0 0   M_a(3,3)*vel(3) 0 -M_a(1,1)*vel(1) ;
        0 0 0  -M_a(2,2)*vel(2) M_a(1,1)*vel(1) 0  ;
        0 -M_a(3,3)*vel(3) M_a(2,2)*vel(2)  0 -M_a(6,6)*vel(6) M_a(5,5)*vel(5) ;
        M_a(3,3)*vel(3) 0 -M_a(1,1)*vel(1)  M_a(6,6)*vel(6) 0 -M_a(4,4)*vel(4) ;
       -M_a(2,2)*vel(2) M_a(1,1)*vel(1) 0   -M_a(5,5)*vel(5) M_a(4,4)*vel(4) 0  ];

% Coreolis matrix
C = C_rb + C_a;

% Restoring forces
g_eta = [ (W-B)*sin(theta);
          -(W-B)*cos(theta)*sin(phi);
          -(W-B)*cos(theta)*cos(phi);
          -(r_g(2)*W-r_b(2)*B)*cos(theta)*cos(phi) + (r_g(3)*W-r_b(3)*B)*cos(theta)*sin(phi);
           (r_g(3)*W-r_b(3)*B)*sin(theta)             + (r_g(1)*W-r_b(1)*B)*cos(theta)*cos(phi)
          -(r_g(1)*W-r_b(1)*B)*cos(theta)*sin(phi) - (r_g(2)*W-r_b(2)*B)*sin(theta)          ];

% Cuadratic Damping matrix
D_cuad = -diag([X_uu*abs(vel(1)) Y_vv*abs(vel(2)) Z_ww*abs(vel(3)) ...
               K_pp*abs(vel(4)) M_qq*abs(vel(5)) N_rr*abs(vel(6))]);

%Damping matrix
Damp = D_lin + D_cuad;

NED_dot = [0;0;0;0;0;0];
% Linear velocities in NED / For a zxy rotation sequence
NED_dot(1) = vel(1)*cos(psi)*cos(theta) + vel(2)*[cos(psi)*sin(theta)*sin(phi)... 
    - sin(psi)*cos(phi)] + vel(3)*[sin(psi)*sin(phi)... 
    + cos(psi)*cos(phi)*sin(theta)];

NED_dot(2) = vel(1)*sin(psi)*cos(theta) + vel(2)*[cos(psi)*cos(phi)... 
    + sin(phi)*sin(theta)*sin(psi)]+ vel(3)*[sin(theta)*sin(psi)*cos(phi)... 
    - cos(psi)*sin(phi)];

NED_dot(3) = -vel(1)*sin(theta) + vel(2)*cos(theta)*sin(phi) + vel(3)*cos(theta)*cos(phi);

%Angular velocities in NED
NED_dot(4) = vel(4) + vel(5)*sin(phi)*tan(theta) + vel(6)*cos(phi)*tan(theta);

NED_dot(5) = vel(5)*cos(phi) - vel(6)*sin(phi);

NED_dot(6) = vel(5)*(sin(phi)/cos(theta)) + vel(6)*(cos(phi)/cos(theta));

vel_dot = M\(tau-(C*vel)-(Damp*vel)-g_eta);

== matlab function comparing_controllers/PD Gravity Compensated Controller/UUV 6DOF Model/Subsystem/MATLAB Function1 ==
  data: tau output; f input; theta input; rx_v input; ry_v input; unused input; rx_h input; ry_h input; rz_h input
function tau = tau_conversion(f, theta, rx_v, ry_v, ~, rx_h, ry_h, rz_h)
tau = [0 0 0 0 0 0].';
tau(1) = (f(1)+f(2)-f(3)-f(4))*cos(theta);
tau(2) = (-f(1)+f(2)-f(3)+f(4))*sin(theta);
tau(3) = -(f(5)+f(6));
tau(4) = (f(6)-f(5))*ry_v + (-f(1)+f(2)-f(3)+f(4))*sin(theta)*rz_h;
tau(5) = (f(6)-f(5))*rx_v + (-f(1)-f(2)+f(3)+f(4))*cos(theta)*rz_h;
tau(6) = (-f(1)+f(2)+f(3)-f(4))*(rx_h*sin(theta)+ry_h*cos(theta));

== matlab function comparing_controllers/PID Controller/6 DOF PID Controller/Thrust allocation/MATLAB Function ==
  data: thrust input; tau output; theta input; rx_v input; ry_v input; unused input; rx_h input; ry_h input; rz_h input
function tau = thrust_conversion(thrust, theta, rx_v, ry_v, ~, rx_h, ry_h, rz_h)
% Errores numericos. El input esta saturado a [100,-100], y estas salidas
% dan valores muchisimo mayores a 35 N c/u
tau = [0 0 0 0 0 0].';
% For surge
s_val = thrust(1)/cos(theta)/4;
tau(1) = tau(1)+s_val;
tau(2) = tau(2)+s_val;
tau(3) = tau(3)-s_val;
tau(4) = tau(4)-s_val;

% For sway
sw_val = thrust(2)/sin(theta)/4;
tau(1) = tau(1)-sw_val;
tau(2) = tau(2)+sw_val;
tau(3) = tau(3)-sw_val;
tau(4) = tau(4)+sw_val;

% For heave
tau(5) = tau(5)+(-thrust(3)/2);
tau(6) = tau(6)+(-thrust(3)/2);

% For yaw
y_val = thrust(6)/(rx_h*sin(theta)+ry_h*cos(theta))/4;
tau(1) = tau(1)-y_val;
tau(2) = tau(2)+y_val;
tau(3) = tau(3)+y_val;
tau(4) = tau(4)-y_val;

% K and M come as zero
% For K
if  thrust(4)~= 0
    %disp("K")
    k_val = (thrust(4)-(-tau(1)+tau(2)-tau(3)+tau(4))*sin(theta)*rz_h)/(2*ry_v);
    tau(5) = tau(5)-k_val;
    tau(6) = tau(6)+k_val;
end

% For M
if thrust(5) ~= 0
    %disp("M")
    M_val = (thrust(5)-(-tau(1)-tau(2)+tau(3)+tau(4))*cos(theta)*rz_h)/(2*rx_v);
    tau(5) = tau(5)-M_val;
    tau(6) = tau(6)+M_val;
end
disp(tau)

== matlab function comparing_controllers/PD Controller/6 DOF PD Controller/Transform/Subsystem2/Rzxy/MATLAB Function1 ==
  data: phi input; Rx output
function Rx = Rx(phi)
Rx = [ 1 0 0;
       0 cos(phi) -sin(phi);
       0 sin(phi) cos(phi); ];

== matlab function comparing_controllers/PID Controller/6 DOF PID Controller/Thrust allocation/MATLAB Function1 ==
  data: tau input; thrust output; alpha input; rx_v input; ry_v input; unused input; rx_h input; ry_h input; rz_h input
function thrust = thrust_allocation(tau, alpha, rx_v, ry_v, ~, rx_h, ry_h, rz_h)
% Mapping matrix
T = [cos(alpha) cos(alpha) -cos(alpha) -cos(alpha) 0 0;
     -sin(alpha) sin(alpha) -sin(alpha) sin(alpha) 0 0;
     0 0 0 0 -1 -1;
     -sin(alpha)*rz_h sin(alpha)*rz_h -sin(alpha)*rz_h sin(alpha)*rz_h -ry_v ry_v;
     -cos(alpha)*rz_h -cos(alpha)*rz_h cos(alpha)*rz_h cos(alpha)*rz_h -rx_v rx_v;
     -(rx_h*sin(alpha)+ry_h*cos(alpha)) (rx_h*sin(alpha)+ry_h*cos(alpha)) (rx_h*sin(alpha)+ry_h*cos(alpha)) -(rx_h*sin(alpha)+ry_h*cos(alpha)) 0 0
    ];
% Control input with Moore–Penrose pseudo-inverse
thrust = pinv(T)*tau;

== matlab function comparing_controllers/PID Controller/6 DOF PID Controller/Transform/Subsystem1/Rzxy/MATLAB Function1 ==
  data: phi input; Rx output
function Rx = Rx(phi)
Rx = [ 1 0 0;
       0 cos(phi) -sin(phi);
       0 sin(phi) cos(phi); ];

== matlab function comparing_controllers/PID Controller/6 DOF PID Controller/Transform/Subsystem1/Rzxy/MATLAB Function2 ==
  data: theta input; Ry output
function Ry = Ry(theta)
Ry = [ cos(theta) 0 sin(theta);
       0          1     0 ;
       -sin(theta) 0 cos(theta); ];

== matlab function comparing_controllers/PID Controller/6 DOF PID Controller/Transform/Subsystem1/Rzxy/MATLAB Function3 ==
  data: psi input; Rz output
function Rz = Rz(psi)
Rz = [ cos(psi) -sin(psi) 0;
       sin(psi) cos(psi)  0;
       0        0         1];

== matlab function comparing_controllers/PID Controller/6 DOF PID Controller/Transform/Subsystem2/Rzxy/MATLAB Function1 ==
  data: phi input; Rx output
function Rx = Rx(phi)
Rx = [ 1 0 0;
       0 cos(phi) -sin(phi);
       0 sin(phi) cos(phi); ];

== matlab function comparing_controllers/PID Controller/6 DOF PID Controller/Transform/Subsystem2/Rzxy/MATLAB Function2 ==
  data: theta input; Ry output
function Ry = Ry(theta)
Ry = [ cos(theta) 0 sin(theta);
       0          1     0 ;
       -sin(theta) 0 cos(theta); ];

== matlab function comparing_controllers/PID Controller/6 DOF PID Controller/Transform/Subsystem2/Rzxy/MATLAB Function3 ==
  data: psi input; Rz output
function Rz = Rz(psi)
Rz = [ cos(psi) -sin(psi) 0;
       sin(psi) cos(psi)  0;
       0        0         1];

== matlab function comparing_controllers/PID Controller/UUV 6DOF Model/+-pi ==
  data: NED input; NED output
function NED = check_angles(NED)
% Correct
if abs(NED(4)) > pi 
    NED(4) = (NED(4)/abs(NED(4)))*(abs(NED(4))-2*pi);
end
if abs(NED(5)) > pi 
    NED(5) = (NED(5)/abs(NED(5)))*(abs(NED(5))-2*pi);
end
if abs(NED(6)) > pi
    NED(6) = (NED(6)/abs(NED(6)))*(abs(NED(6))-2*pi);
    disp((NED(6)/abs(NED(6)))*(abs(NED(6))-2*pi))
end

== matlab function comparing_controllers/PID Controller/UUV 6DOF Model/MATLAB Function ==
  data: vel_dot output; tau input; vel input; phi input; theta input; NED_dot output; psi input
function [vel_dot,NED_dot]= UUV_forward_dynamics(tau,vel,phi,theta,psi)
% Skew symmetric matrix
S = @(s) [0    -s(3) s(2);
          s(3) 0     -s(1);
          -s(2) s(1)  0    ];  

% Vehicle parameters
m = 24;
vol = 0.02306187;
W = m*9.81;
B = W*1.005; %1000*9.81*vol;

r_g = [0 0 0].';    % Distance from origin to center of mass
r_b = [0 0 -0.10726].';    % Distance from origin to center of buoyancy
I_g = [0.900121387  -0.000186482 0.0072251;
       -0.000186482 1.754494427  0.020319615;
       0.0072251    0.020319615  1.43389     ]; % Rigid-body inertia matrix

% Rigid-Body Inertia Matrix
M_rb = [ m*eye(3)    -m*S(r_g);
         m*S(r_g)         I_g ];

% Added mass matrix
M_a = diag([16.8374 20.2748 35.3180 0.2165 0.6869 0.6157]);

% Mass matrix
M = M_rb + M_a;

% Linear damping coefficients
X_u = -0.3431;
Y_v = 0.0518;
Z_w = -0.5841;
K_p = 0.0064;
M_q = 0.04;
N_r = -0.1063;

D_lin = -diag([X_u Y_v Z_w K_p M_q N_r]);

% Cuadratic damping coefficients
X_uu = -111.7397;
Y_vv = -44.4058;
Z_ww = -157.1951;
K_pp = -0.4634;
M_qq = -0.2902;
N_rr = -2.2897;

%------------ UUV dynamic model parametrization ----------------%
% Rigid-body Coriolis-centripetal Matrix
C_rb = [ zeros(3)             -m*S(vel(1:3))-m*S(vel(4:6))*S(r_g);
        -m*S(vel(1:3))+m*S(r_g)*S(vel(4:6))            -S(I_g*vel(4:6))];

% Coreolis added mass matrix 
C_a = [ 0 0 0   0 -M_a(3,3)*vel(3) M_a(2,2)*vel(2) ;
        0 0 0   M_a(3,3)*vel(3) 0 -M_a(1,1)*vel(1) ;
        0 0 0  -M_a(2,2)*vel(2) M_a(1,1)*vel(1) 0  ;
        0 -M_a(3,3)*vel(3) M_a(2,2)*vel(2)  0 -M_a(6,6)*vel(6) M_a(5,5)*vel(5) ;
        M_a(3,3)*vel(3) 0 -M_a(1,1)*vel(1)  M_a(6,6)*vel(6) 0 -M_a(4,4)*vel(4) ;
       -M_a(2,2)*vel(2) M_a(1,1)*vel(1) 0   -M_a(5,5)*vel(5) M_a(4,4)*vel(4) 0  ];

% Coreolis matrix
C = C_rb + C_a;

% Restoring forces
g_eta = [ (W-B)*sin(theta);
          -(W-B)*cos(theta)*sin(phi);
          -(W-B)*cos(theta)*cos(phi);
          -(r_g(2)*W-r_b(2)*B)*cos(theta)*cos(phi) + (r_g(3)*W-r_b(3)*B)*cos(theta)*sin(phi);
           (r_g(3)*W-r_b(3)*B)*sin(theta)             + (r_g(1)*W-r_b(1)*B)*cos(theta)*cos(phi)
          -(r_g(1)*W-r_b(1)*B)*cos(theta)*sin(phi) - (r_g(2)*W-r_b(2)*B)*sin(theta)          ];

% Cuadratic Damping matrix
D_cuad = -diag([X_uu*abs(vel(1)) Y_vv*abs(vel(2)) Z_ww*abs(vel(3)) ...
               K_pp*abs(vel(4)) M_qq*abs(vel(5)) N_rr*abs(vel(6))]);

%Damping matrix
Damp = D_lin + D_cuad;

NED_dot = [0;0;0;0;0;0];
% Linear velocities in NED / For a zxy rotation sequence
NED_dot(1) = vel(1)*cos(psi)*cos(theta) + vel(2)*[cos(psi)*sin(theta)*sin(phi)... 
    - sin(psi)*cos(phi)] + vel(3)*[sin(psi)*sin(phi)... 
    + cos(psi)*cos(phi)*sin(theta)];

NED_dot(2) = vel(1)*sin(psi)*cos(theta) + vel(2)*[cos(psi)*cos(phi)... 
    + sin(phi)*sin(theta)*sin(psi)]+ vel(3)*[sin(theta)*sin(psi)*cos(phi)... 
    - cos(psi)*sin(phi)];

NED_dot(3) = -vel(1)*sin(theta) + vel(2)*cos(theta)*sin(phi) + vel(3)*cos(theta)*cos(phi);

%Angular velocities in NED
NED_dot(4) = vel(4) + vel(5)*sin(phi)*tan(theta) + vel(6)*cos(phi)*tan(theta);

NED_dot(5) = vel(5)*cos(phi) - vel(6)*sin(phi);

NED_dot(6) = vel(5)*(sin(phi)/cos(theta)) + vel(6)*(cos(phi)/cos(theta));

vel_dot = M\(tau-(C*vel)-(Damp*vel)-g_eta);

== matlab function comparing_controllers/PD Controller/UUV 6DOF Model/+-pi ==
  data: NED input; NED output
function NED = check_angles(NED)
% Correct
if abs(NED(4)) > pi 
    NED(4) = (NED(4)/abs(NED(4)))*(abs(NED(4))-2*pi);
end
if abs(NED(5)) > pi 
    NED(5) = (NED(5)/abs(NED(5)))*(abs(NED(5))-2*pi);
end
if abs(NED(6)) > pi
    NED(6) = (NED(6)/abs(NED(6)))*(abs(NED(6))-2*pi);
    disp((NED(6)/abs(NED(6)))*(abs(NED(6))-2*pi))
end

== matlab function comparing_controllers/PID Controller/UUV 6DOF Model/Subsystem/MATLAB Function1 ==
  data: tau output; f input; theta input; rx_v input; ry_v input; unused input; rx_h input; ry_h input; rz_h input
function tau = tau_conversion(f, theta, rx_v, ry_v, ~, rx_h, ry_h, rz_h)
tau = [0 0 0 0 0 0].';
tau(1) = (f(1)+f(2)-f(3)-f(4))*cos(theta);
tau(2) = (-f(1)+f(2)-f(3)+f(4))*sin(theta);
tau(3) = -(f(5)+f(6));
tau(4) = (f(6)-f(5))*ry_v + (-f(1)+f(2)-f(3)+f(4))*sin(theta)*rz_h;
tau(5) = (f(6)-f(5))*rx_v + (-f(1)-f(2)+f(3)+f(4))*cos(theta)*rz_h;
tau(6) = (-f(1)+f(2)+f(3)-f(4))*(rx_h*sin(theta)+ry_h*cos(theta));

== matlab function comparing_controllers/Computed Torque/Computed Torque Controller/6 PD + fb linearization Controllers/MATLAB Function ==
  data: M output; in input
function M = M(in)
% Skew symmetric matrix
S = @(s) [0    -s(3) s(2);
          s(3) 0     -s(1);
          -s(2) s(1)  0    ];  

% Vehicle parameters
m = 24;

r_g = [0 0 0].';    % Distance from origin to center of mass
I_g = [0.900121387  -0.000186482 0.0072251;
       -0.000186482 1.754494427  0.020319615;
       0.0072251    0.020319615  1.43389     ]; % Rigid-body inertia matrix

% Rigid-Body Inertia Matrix
M_rb = [ m*eye(3)    -m*S(r_g);
         m*S(r_g)         I_g ];

% Added mass matrix
M_a = diag([16.8374 20.2748 35.3180 0.2165 0.6869 0.6157]);

% Mass matrix
M = (M_rb + M_a)*in;
